simulink model "clik_inverse"  (R2022b)
settings: Solver=ode1  StartTime=0.0  StopTime=4  FixedStep=0.001  RelTol=1e-3
undefined symbols (not defined in the file or in its folder): DiscIntNeverNeededParam, Tc
settings Model: Creator=Xp  LastModifiedBy=shubham
settings SolverCC: AlgebraicLoopSolver=TrustRegion
settings DataIOCC: LimitDataPoints=on  SaveFormat=Array  SignalLoggingSaveFormat=ModelDataLogs  ReturnWorkspaceOutputs=off
settings OptimizationCC: ExpressionDepthLimit=2147483647  InitFltsAndDblsToZero=on  LifeSpan=inf
settings DebuggingCC: SaveWithParameterizedLinksMsg=none  UnderspecifiedInitializationDetection=Classic  MergeDetectMultiDrivingBlocksExec=none  SolverPrmCheckMsg=warning  MultiTaskDSMMsg=warning  MultiTaskCondExecSysMsg=none  FcnCallInpInsideContextMsg=warning  UnconnectedInputMsg=warning  UnconnectedOutputMsg=warning  UnconnectedLineMsg=warning  StateNameClashWarn=warning  SFUnexpectedBacktrackingDiag=warning  SFNoUnconditionalDefaultTransitionDiag=warning  SFExecutionAtInitializationDiag=none  SFMachineParentedDataDiag=warning  ArithmeticOperatorsInVariantConditions=warning
settings HardwareCC: ProdBitPerPointer=32  ProdBitPerSizeT=32  ProdBitPerPtrDiffT=32  ProdLargestAtomicFloat=None  ProdIntDivRoundTo=Undefined  ProdEndianess=Unspecified  ProdWordSize=32  ProdHWDeviceType=32-bit Generic
settings ModelReferenceCC: EnableRefExpFcnMdlSchedulingChecks=on  PropagateSignalLabelsOutOfModel=off
settings SFSimCC: CustomCodeUndefinedFunction=UseInterfaceOnly
settings RTWCC: DLArmComputeVersion=19.05
settings CodeAppCC: StateflowObjectComments=on
settings GRTTargetCC: TargetLangStandard=C89/C90 (ANSI)  CombineOutputUpdateFcns=off  GRTInterface=on
settings ConfigComp: CovMetricSettings=dw  CovSaveCumulativeToWorkspaceVar=on  CovSaveSingleToWorkspaceVar=on

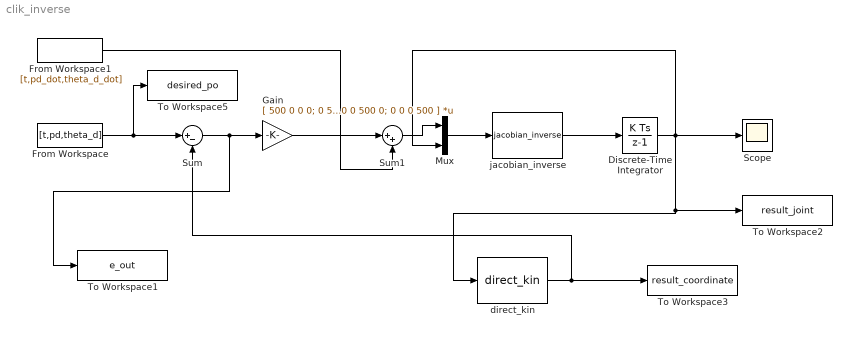
== system clik_inverse ==
  Discrete-Time Integrator : DiscreteIntegrator  InitialCondition=|  SampleTime=Tc  ICPrevOutput=DiscIntNeverNeededParam  ICPrevScaledInput=DiscIntNeverNeededParam
      | [-0.927;
      | -1.287;
      | 0.70; 2.2143]
  From Workspace : FromWorkspace  VariableName=[t,pd,theta_d]  SampleTime=Tc
  From Workspace1 : FromWorkspace  VariableName=[t,pd_dot,theta_d_dot]  SampleTime=Tc
  Gain : Gain  Gain=[ 500 0 0 0; 0 500 0 0; 0 0 500 0; 0 0 0 500 ]  Multiplication=Matrix(K*u)
  Mux : Mux  Inputs=2
  Scope : Scope
  Sum : Sum  Inputs=|+-
  Sum1 : Sum  Inputs=|++
  To Workspace1 : ToWorkspace  VariableName=e_out  SampleTime=-1
  To Workspace2 : ToWorkspace  VariableName=result_joint  SampleTime=-1
  To Workspace3 : ToWorkspace  VariableName=result_coordinate  SampleTime=-1
  To Workspace5 : ToWorkspace  VariableName=desired_po  SaveFormat=Timeseries  SampleTime=-1
  direct_kin : MATLABFcn  Description=call direct_kin.m  MATLABFcn=direct_kin  OutputDimensions=4  OutputSignalType=real
  jacobian_inverse : MATLABFcn  MATLABFcn=jacobian_inverse  OutputDimensions=4  OutputSignalType=real
  wires:
  Sum/1 -> To Workspace1/1, Gain/1
  Sum1/1 -> Mux/1
  Gain/1 -> Sum1/1
  direct_kin/1 -> To Workspace3/1, Sum/2
  jacobian_inverse/1 -> Discrete-Time Integrator/1
  Discrete-Time Integrator/1 -> direct_kin/1, To Workspace2/1, Scope/1, Mux/2
  From Workspace1/1 -> Sum1/2
  Mux/1 -> jacobian_inverse/1
  From Workspace/1 -> To Workspace5/1, Sum/1
